simulink model "PMSM_PI_decomposition"  (R2024a)
settings: Solver=VariableStepAuto  StartTime=0.0  StopTime=5  FixedStep=0.000025  RelTol=1e-4  EnableMultiTasking=on
InitFcn:
  | Ts = 10e-6;
  | 
  | R = 0.958;
  | Ld = 5.25e-3;
  | Lq = 12e-3;
  | Pn = 4;
  | flux = 0.1827;
values from neighbouring files (symbols this model uses):
  A = [0, -1; 0, -Rs/Lq]    [StateSpace.m]    (also in untitled.m = [0 1; -100 -5])
  Flux = 0.1827    [Parameters.m]    (also in StateSpace.m = 0.192)
  Ki = (Ld*2*pi*fsw)/10    (= 2.4975661596)    [StateSpace.m]
  Kp = (Lq*2*pi*fsw)/10    (= 2.4975661596)    [StateSpace.m]
  L_d = 0.00525    [Parameters.m]
  L_q = 0.00525    [Parameters.m]
  p = 4    [Parameters.m]    (also in StateSpace.m)
  R_s = 0.9585    [Parameters.m]
libraries: mcbcontrolslib x2, spsDCVoltageSourceLib x1, mcbhdlpositiondecoderlib x1, spsPermanentMagnetSynchronousMachineLib x1, spsSVPWMGenerator2LevelLib x1, simulink x1, spsUniversalBridgeLib x1, sps_lib x1
settings Model: Creator=SUN  LastModifiedBy=didad
settings SolverCC: InitialStep=0.0002  ZeroCrossControl=DisableAll  AlgebraicLoopSolver=TrustRegion
settings DataIOCC: LimitDataPoints=on  SaveFormat=Array  SignalLoggingSaveFormat=ModelDataLogs  ReturnWorkspaceOutputs=off
settings OptimizationCC: ExpressionDepthLimit=2147483647  InitFltsAndDblsToZero=on  LifeSpan=inf
settings DebuggingCC: UnderspecifiedInitializationDetection=Classic  MergeDetectMultiDrivingBlocksExec=none  SolverPrmCheckMsg=warning  FcnCallInpInsideContextMsg=warning  UnconnectedInputMsg=warning  UnconnectedOutputMsg=warning  UnconnectedLineMsg=warning  StateNameClashWarn=warning  SFUnexpectedBacktrackingDiag=warning  SFNoUnconditionalDefaultTransitionDiag=warning  SFExecutionAtInitializationDiag=none  ArithmeticOperatorsInVariantConditions=warning
settings HardwareCC: ProdBitPerPointer=32  ProdBitPerSizeT=32  ProdBitPerPtrDiffT=32  ProdLargestAtomicFloat=None  ProdIntDivRoundTo=Undefined  ProdEndianess=Unspecified  ProdWordSize=32  ProdHWDeviceType=32-bit Generic
settings ModelReferenceCC: EnableRefExpFcnMdlSchedulingChecks=on  PropagateSignalLabelsOutOfModel=off
settings SFSimCC: SimUseLocalCustomCode=off  CustomCodeUndefinedFunction=UseInterfaceOnly
settings RTWCC: RTWUseLocalCustomCode=off  GPUComputeCapability=3.5
settings CodeAppCC: StateflowObjectComments=on
settings GRTTargetCC: TargetLangStandard=C89/C90 (ANSI)  CombineOutputUpdateFcns=off  GRTInterface=on
settings ConfigComp: CovMetricSettings=dw  CovSaveCumulativeToWorkspaceVar=on  CovSaveSingleToWorkspaceVar=on  CovExternalEMLEnable=off  CovSFcnEnable=off
settings SimscapeCC: SimscapeNormalizeSystem=off

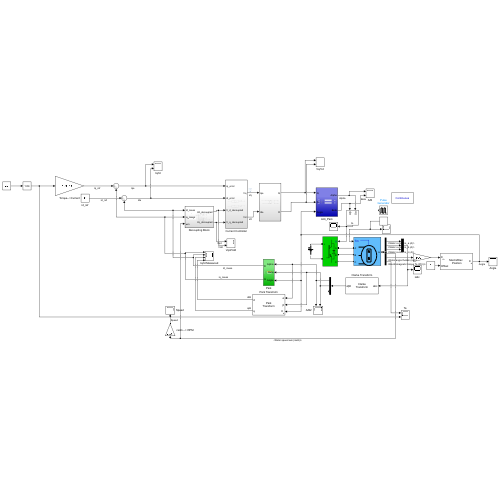
[thumbnail: Simulink's stored preview of the top-level diagram]
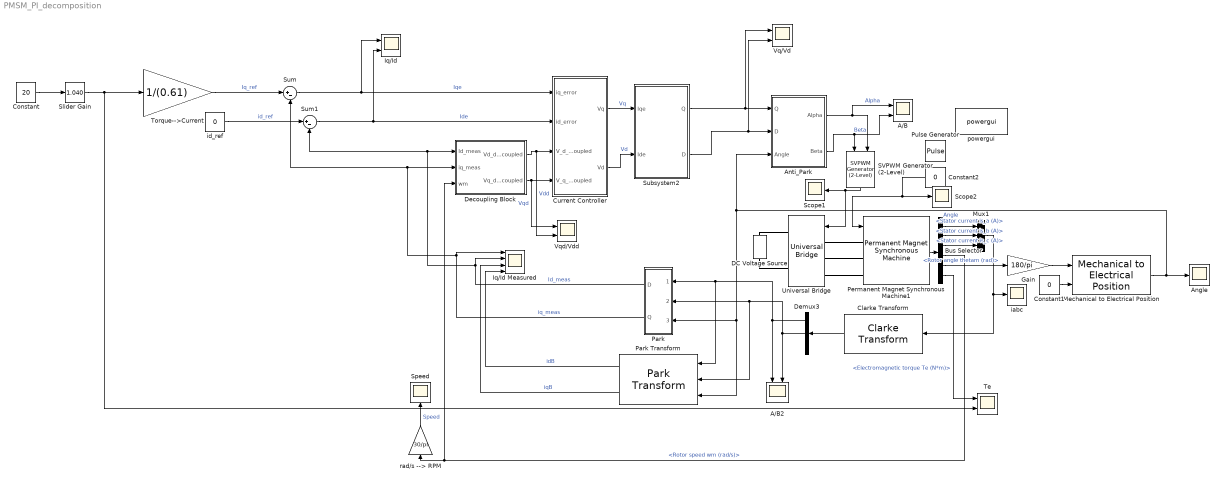
== system PMSM_PI_decomposition ==
  A/B : Scope  NumInputPorts=2
  A/B2 : Scope  NumInputPorts=2
  Angle : Scope
  Anti_Park : Subsystem
  Bus Selector : BusSelector  OutputSignals=Stator current is_a (A),Stator current is_b (A),Stator current is_c (A),Rotor speed wm (rad/s),Rotor angle thetam (rad),Electromagnetic torque Te (N*m)
  Clarke Transform : mcbcontrolslib/Clarke Transform  VariantControl=Variant2  PhaseInput=Three inputs  EnPowerInv=off
      settings: LibrarySourceBlock=mcblib/Controls/Math Transforms/Clarke Transform
  Constant : Constant  Value=20
  Constant1 : Constant  Value=0
  Constant2 : Constant  Value=0
  Current Controller : Subsystem
  DC Voltage Source : spsDCVoltageSourceLib/DC Voltage Source  Amplitude=100  Measurements=None
  Decoupling Block : Subsystem
  Demux3 : Demux  Outputs=3
  Gain : Gain  Gain=180/pi
  Iq/Id : Scope  NumInputPorts=2
  Iq/Id Measured : Scope  NumInputPorts=4
  Mechanical to Electrical Position : mcbhdlpositiondecoderlib/Mechanical to Electrical Position  PolePairsInputType=Specify via dialog  NrPP=4  selectedRange=Degrees  MechOfstInputType=Input port  mechOffsetIn=0  maxAngleIn=360  InputDataType=single  VariantSelect=floating-point
      settings: LibrarySourceBlock=mcbhdllib/Sensor Decoders/Mechanical to Electrical Position
  Mux1 : Mux  Inputs=3
  Park : Subsystem
  Park Transform : mcbcontrolslib/Park Transform  PhaseInput=Two inputs  AxisAlignment=D-axis  ThetaInput=Electrical position  AngleInput=Degrees  N_points=1024
      settings: LibrarySourceBlock=mcblib/Controls/Math Transforms/Park Transform
  Permanent Magnet Synchronous Machine1 : spsPermanentMagnetSynchronousMachineLib/Permanent Magnet Synchronous Machine  NbPhases=3  FluxDistribution=Sinusoidal  RotorType=Round  MechanicalLoad=Torque Tm  PresetModel=No  ShowDetailedParameters=on  MeasurementBus=off  Resistance=R_s  Inductance=8.5e-3  dqInductances=[5.25e-3,12e-3]  La=L_d  MachineConstant=Torque Constant (N.m / A_peak)  Flux=0.10167  VoltageCst=73.7612  TorqueCst=0.61  Flat=120  Mechanical=[0.002521 0.04793 4]  PolePairs=4  InitialConditions=[0,0, 0,0]  InitialConditions5ph=[0 0 0 0 0 0]  RefAngle=90 degrees behind phase A axis (modified Park)  IterativeDiscreteModel=Trapezoidal non iterative  TsBlock=-1  TsPowergui=0
  Pulse Generator : DiscretePulseGenerator  PulseType=Time based  Amplitude=10  Period=1  PulseWidth=5
  SVPWM Generator (2-Level) : spsSVPWMGenerator2LevelLib/SVPWM Generator (2-Level)  InputType=alpha-beta components  SwitchingPattern=Pattern #1  Fc=2000  ParUref=[0.8 -30 50]  Ts=0
  Scope1 : Scope
  Scope2 : Scope
  Slider Gain : simulink/Math Operations/Slider Gain  gain=1.040  low=0  high=2
  Speed : Scope
  Subsystem2 : Subsystem
  Sum : Sum  Inputs=|+-
  Sum1 : Sum  Inputs=|+-
  Te : Scope  NumInputPorts=2
  Torque-->Current : Gain  Gain=1/(0.61)
  Universal Bridge : spsUniversalBridgeLib/Universal Bridge  Arms=3  SnubberResistance=0.01  SnubberCapacitance=inf  Device=IGBT / Diodes  Ron=1e-3  Lon=0  ForwardVoltages="[  0  0  ]"  ForwardVoltage=0  GTOparameters=[ 10e-6 , 20e-6 ]  IGBTparameters=[ 1e-6 , 2e-6 ]  Measurements=None  Measurements_2=None  converterType=Rectifier
  Vq/Vd : Scope  NumInputPorts=2
  Vqd/Vdd : Scope  NumInputPorts=2
  iabc : Scope
  id_ref : Constant  Value=0
  powergui : sps_lib/powergui  Priority=1  SimulationMode=Continuous  SampleTime=50e-6  frequency=60  Iterations=50  frequencyindice=0  Pbase=100e6  ErrMax=1e-4  UnitsV=kV  UnitsW=MW  buscounter=0  FunctionMessages=off  echomessages=off  EnableUseOfTLC=off  CurrentSourceSwitches=off  DisableSnubberDevices=off  DisableRonSwitches=off  DisableVfSwitches=off  DisplayEquations=off  AutomaticDiscreteSolvers=off  SolverType=Tustin/Backward Euler (TBE)  Interpol=off  ExternalGateDelay=off  methode=off  Ts=100  x0status=blocks  SPID=on  SwTol=0  HookPort=off  NonlinearTolerance=1e-4  nMaxIteration=100  ContinueOnMaxIteration=off  RestoreLinks=warning  ResistiveCurrentMeasurement=off  Frange=[0:2:500]  Ylog=off  Xlog=on  ShowGrid=off  save=off  variable=ZData  structure=0  ZoomFFT=off  StartTime=0.0  cycles=1  DisplayStyle=1  fundamental=60  FreqAxis=off  MaxFrequency=1000  frequencyindicesteady=1  RmsSteady=1  display=off
  rad/s --> RPM : Gain  Gain=30/pi
  wires:
  Constant2/1 -> Permanent Magnet Synchronous Machine1/1, Scope2/1
  Anti_Park/2(Beta) -> A/B/2, SVPWM Generator (2-Level)/2  "Beta"
  Bus Selector/3 -> Mux1/3  "<Stator current is_c (A)>"
  Bus Selector/2 -> Mux1/2  "<Stator current is_b (A)>"
  Bus Selector/1 -> Mux1/1  "<Stator current is_a (A)>"
  Permanent Magnet Synchronous Machine1/1 -> Bus Selector/1
  Bus Selector/6 -> Te/1  "<Electromagnetic torque Te (N*m)>"
  id_ref/1 -> Sum1/1  "id_ref"
  Sum/1 -> Current Controller/1(iq_error), Iq/Id/1  "Iqe"
  Park/2(Q) -> Sum/2, Decoupling Block/2(iq_meas), Iq/Id Measured/1  "iq_meas"
  Torque-->Current/1 -> Sum/1  "Iq_ref"
  Slider Gain/1 -> Te/2, Torque-->Current/1
  Park/1(D) -> Iq/Id Measured/2, Sum1/2, Decoupling Block/1(Id_meas)  "Id_meas"
  Sum1/1 -> Current Controller/2(id_error), Iq/Id/2  "Ide"
  Bus Selector/4 -> Decoupling Block/3(wm), rad/s --> RPM/1  "<Rotor speed wm (rad/s)>"
  Mux1/1 -> Clarke Transform/1, iabc/1
  rad/s --> RPM/1 -> Speed/1  "Speed"
  Demux3/1 -> A/B2/1, Park Transform/1, Park/1(Alpha)
  Demux3/2 -> A/B2/2, Park Transform/2, Park/2(Beta)
  Bus Selector/5 -> Gain/1  "<Rotor angle thetam (rad)>"
  Mechanical to Electrical Position/1 -> Park Transform/3, Park/3(Angle), Anti_Park/3(Angle), Angle/1  "Angle"
  Constant1/1 -> Mechanical to Electrical Position/2
  Decoupling Block/1(Vd_decoupled) -> Vqd/Vdd/2, Current Controller/3(V_d_decoupled)  "Vdd"
  Decoupling Block/2(Vq_decoupled) -> Vqd/Vdd/1, Current Controller/4(V_q_decoupled)  "Vqd"
  Constant/1 -> Slider Gain/1
  SVPWM Generator (2-Level)/1 -> Universal Bridge/1, Scope1/1
  Anti_Park/1(Alpha) -> SVPWM Generator (2-Level)/1, A/B/1  "Alpha"
  Subsystem2/2(D) -> Vq/Vd/2, Anti_Park/2(D)
  Current Controller/2(Vd) -> Subsystem2/2(Ide)  "Vd"
  Current Controller/1(Vq) -> Subsystem2/1(Iqe)  "Vq"
  Subsystem2/1(Q) -> Vq/Vd/1, Anti_Park/1(Q)
  Clarke Transform/1 -> Demux3/1
  Gain/1 -> Mechanical to Electrical Position/1
  Park Transform/1 -> Iq/Id Measured/4  "idB"
  Park Transform/2 -> Iq/Id Measured/3  "iqB"
  connections:
  Universal Bridge/LConn1 -- Permanent Magnet Synchronous Machine1/LConn1
  Universal Bridge/LConn2 -- Permanent Magnet Synchronous Machine1/LConn2
  Universal Bridge/LConn3 -- Permanent Magnet Synchronous Machine1/LConn3
  Universal Bridge/RConn1 -- DC Voltage Source/RConn1
  DC Voltage Source/LConn1 -- Universal Bridge/RConn2

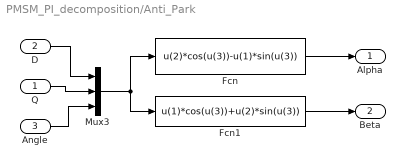
== system PMSM_PI_decomposition/Anti_Park ==
  Q : Inport
  D : Inport  Port=2
  Angle : Inport  Port=3
  Fcn : Fcn  Expr=u(2)*cos(u(3))-u(1)*sin(u(3))
  Fcn1 : Fcn  Expr=u(1)*cos(u(3))+u(2)*sin(u(3))
  Mux3 : Mux  Inputs=3
  Alpha : Outport  VectorParamsAs1DForOutWhenUnconnected=off
  Beta : Outport  Port=2  VectorParamsAs1DForOutWhenUnconnected=off
  wires:
  Angle/1 -> Mux3/3
  Fcn1/1 -> Beta/1
  Mux3/1 -> Fcn1/1, Fcn/1
  Fcn/1 -> Alpha/1
  D/1 -> Mux3/1
  Q/1 -> Mux3/2

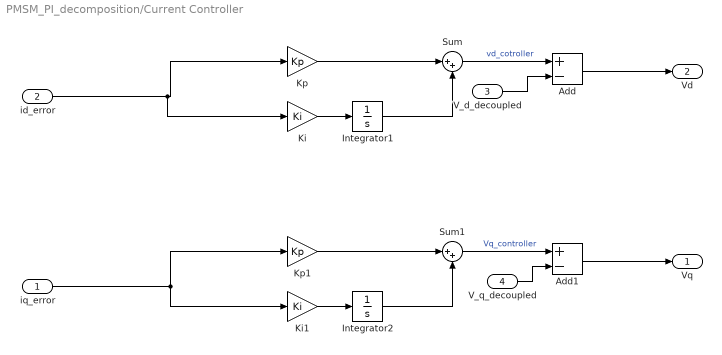
== system PMSM_PI_decomposition/Current Controller ==
  iq_error : Inport
  id_error : Inport  Port=2
  V_d_decoupled : Inport  Port=3
  V_q_decoupled : Inport  Port=4
  Add : Sum  Inputs=+-
  Add1 : Sum  Inputs=+-
  Integrator1 : Integrator
  Integrator2 : Integrator
  Ki : Gain  Gain=Ki
  Ki1 : Gain  Gain=Ki
  Kp : Gain  Gain=Kp
  Kp1 : Gain  Gain=Kp
  Sum : Sum  Inputs=|++
  Sum1 : Sum  Inputs=|++
  Vq : Outport
  Vd : Outport  Port=2
  wires:
  V_q_decoupled/1 -> Add1/2
  Ki1/1 -> Integrator2/1
  V_d_decoupled/1 -> Add/2
  Kp1/1 -> Sum1/1
  Integrator2/1 -> Sum1/2
  Integrator1/1 -> Sum/2
  Ki/1 -> Integrator1/1
  Kp/1 -> Sum/1
  Sum/1 -> Add/1  "vd_cotroller"
  Sum1/1 -> Add1/1  "Vq_controller"
  Add/1 -> Vd/1
  Add1/1 -> Vq/1
  id_error/1 -> Ki/1, Kp/1
  iq_error/1 -> Ki1/1, Kp1/1

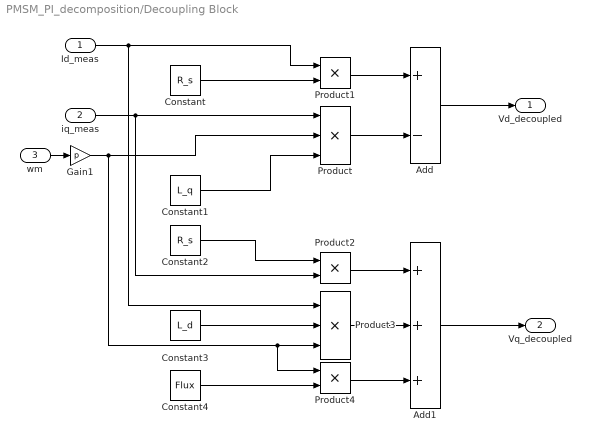
== system PMSM_PI_decomposition/Decoupling Block ==
  Id_meas : Inport
  iq_meas : Inport  Port=2
  wm : Inport  Port=3
  Add : Sum  Inputs=+-
  Add1 : Sum  Inputs=+++
  Constant : Constant  Value=R_s
  Constant1 : Constant  Value=L_q
  Constant2 : Constant  Value=R_s
  Constant3 : Constant  Value=L_d
  Constant4 : Constant  Value=Flux
  Gain1 : Gain  Gain=p
  Product : Product  Inputs=3
  Product1 : Product
  Product2 : Product
  Product3 : Product  Inputs=3
  Product4 : Product
  Vd_decoupled : Outport
  Vq_decoupled : Outport  Port=2
  wires:
  Add/1 -> Vd_decoupled/1
  Product1/1 -> Add/1
  Constant/1 -> Product1/2
  Id_meas/1 -> Product1/1, Product3/1
  Product/1 -> Add/2
  Gain1/1 -> Product4/1, Product3/3, Product/2
  Constant1/1 -> Product/3
  Add1/1 -> Vq_decoupled/1
  Product2/1 -> Add1/1
  Constant2/1 -> Product2/1
  iq_meas/1 -> Product/1, Product2/2
  Product3/1 -> Add1/2
  Constant3/1 -> Product3/2
  Product4/1 -> Add1/3
  Constant4/1 -> Product4/2
  wm/1 -> Gain1/1

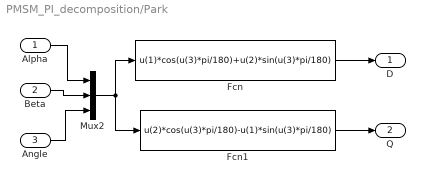
== system PMSM_PI_decomposition/Park ==
  Alpha : Inport
  Beta : Inport  Port=2
  Angle : Inport  Port=3
  Fcn : Fcn  Expr=u(1)*cos(u(3)*pi/180)+u(2)*sin(u(3)*pi/180)
  Fcn1 : Fcn  Expr=u(2)*cos(u(3)*pi/180)-u(1)*sin(u(3)*pi/180)
  Mux2 : Mux  Inputs=3
  D : Outport  VectorParamsAs1DForOutWhenUnconnected=off
  Q : Outport  Port=2  VectorParamsAs1DForOutWhenUnconnected=off
  wires:
  Beta/1 -> Mux2/2
  Mux2/1 -> Fcn1/1, Fcn/1
  Angle/1 -> Mux2/3
  Alpha/1 -> Mux2/1
  Fcn1/1 -> Q/1
  Fcn/1 -> D/1

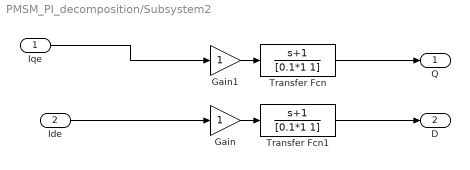
== system PMSM_PI_decomposition/Subsystem2 ==
  Iqe : Inport
  Ide : Inport  Port=2
  Gain : Gain
  Gain1 : Gain
  Transfer Fcn : TransferFcn  Numerator=[1 1]  Denominator=[0.1*1 1]
  Transfer Fcn1 : TransferFcn  Numerator=[1 1]  Denominator=[0.1*1 1]
  Q : Outport
  D : Outport  Port=2
  wires:
  Gain1/1 -> Transfer Fcn/1
  Ide/1 -> Gain/1
  Gain/1 -> Transfer Fcn1/1
  Iqe/1 -> Gain1/1
  Transfer Fcn/1 -> Q/1
  Transfer Fcn1/1 -> D/1
